simulink model "IIR122parallel"  (Simulink 7.9)
settings: Solver=FixedStepDiscrete  StartTime=0.0  StopTime=10.0  RelTol=1e-3
values from neighbouring files (symbols this model uses):
  G = 3/4    (= 0.75)    [IIRFrequencyResponse.m]    (also in createFIR.m = 0.25; createIIR.m; lab122freqresponseIIR.m)
libraries: dspsigops x2
settings Model: Creator=llugos  LastModifiedBy=llugos

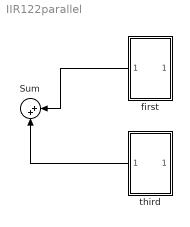
== system IIR122parallel ==
  Sum : Sum  Inputs=|++
  first : Subsystem
  third : Subsystem
  wires:
  first/1(Out1) -> Sum/1
  third/1(Out1) -> Sum/2

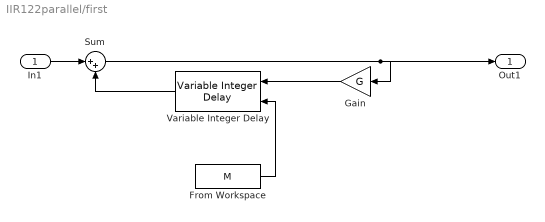
== system IIR122parallel/first ==
  In1 : Inport
  From Workspace : FromWorkspace  VariableName=M  SampleTime=0
  Gain : Gain  Gain=G
  Sum : Sum  Inputs=|++
  Variable Integer Delay : dspsigops/Variable Integer Delay  dmax=100  InputProcessing=Columns as channels (frame based)  ic=0  noDFT=off
  Out1 : Outport
  wires:
  Gain/1 -> Variable Integer Delay/1
  From Workspace/1 -> Variable Integer Delay/2
  Variable Integer Delay/1 -> Sum/2
  Sum/1 -> Gain/1, Out1/1
  In1/1 -> Sum/1

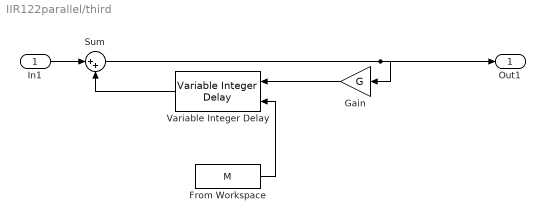
== system IIR122parallel/third ==
  In1 : Inport
  From Workspace : FromWorkspace  VariableName=M  SampleTime=0
  Gain : Gain  Gain=G
  Sum : Sum  Inputs=|++
  Variable Integer Delay : dspsigops/Variable Integer Delay  dmax=100  InputProcessing=Columns as channels (frame based)  ic=0  noDFT=off
  Out1 : Outport
  wires:
  Gain/1 -> Variable Integer Delay/1
  From Workspace/1 -> Variable Integer Delay/2
  Variable Integer Delay/1 -> Sum/2
  Sum/1 -> Gain/1, Out1/1
  In1/1 -> Sum/1
